simulink library "uavsimBlockset_Cularis"  (R2014b)
settings: Solver=ode45  StartTime=0.0  StopTime=10.0  RelTol=1e-3
undefined symbols (not defined in the file): aircraftmask_originNED_ECEF_rrm, aircraftmask_p0_NED_m, aircraftmask_phithetapsi0, aircraftmask_pqr0, aircraftmask_uvw0, fflib_degdegm2rrm, flat2lla, uavsim
libraries: uavsimBlockset_ServoHS55 x4, simulink_extras x1, uavsimBlockset_Cularis_Aerandpropulsion x1, uavsimblockset_SixDOFKinematics x1
settings Model: Creator=mstolle  LastModifiedBy=j.bolting

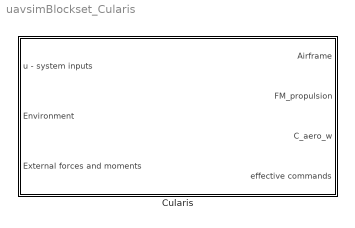
== system uavsimBlockset_Cularis ==
  Cularis : Subsystem  mask{mask_zagi_phithetapsi0=aircraftmask_phithetapsi0, mask_zagi_p0_ECEF_lla=fflib_degdegm2rrm(flat2lla(aircraftmask_p0_NED_m, rad2deg(aircraftmask_originNED_ECEF_rrm(1:2)), 0, aircraftmask_originNED_ECEF_rrm(3))), mask_zagi_originNED_ECEF_rrm=aircraftmask_originNED_ECEF_rrm, mask_zagi_pqr0=aircraftmask_pqr0, mask_zagi_uvw0=aircraftmask_uvw0, uavsim=uavsim}
      mask prompts: mask_zagi_phithetapsi0 "Initial euler angles [rad]"; mask_zagi_p0_ECEF_lla "Initial position ECEF [rad rad m]"; mask_zagi_originNED_ECEF_rrm "Origin NED frame, ECEF-WGS84, [rad rad m]"; mask_zagi_pqr0 "Initial body rotation rates [rad/s]"; mask_zagi_uvw0 "Initial velocity body frame [m/s]"; uavsim "Parameter set"
      mask Display: image(imread('images/cularis.png'),[.3, .3, .4, .4])

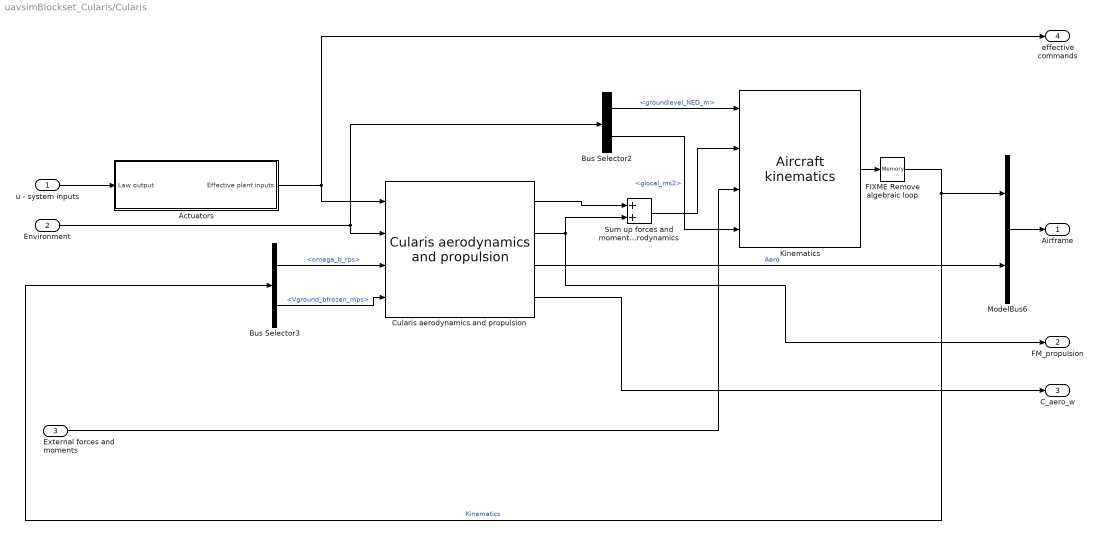
== system uavsimBlockset_Cularis/Cularis ==
  u - system inputs : Inport  OutDataTypeStr=Bus: CMD
  Environment : Inport  Port=2  OutDataTypeStr=Bus: Environment
  External forces and moments : Inport  Port=3
  Actuators : Subsystem  TreatAsAtomicUnit=on
  Bus Selector2 : BusSelector  OutputSignals=groundlevel_NED_m,glocal_ms2
  Bus Selector3 : BusSelector  OutputSignals=RotationalVelocity.omega_b_rps,Velocity.Vground_bfrozen_mps
  Cularis aerodynamics and propulsion : uavsimBlockset_Cularis_Aerandpropulsion/Cularis aerodynamics and propulsion  SystemSampleTime=-1
  FIXME Remove algebraic loop : Memory  X0=1e-6
  Kinematics : uavsimblockset_SixDOFKinematics/Aircraft kinematics  mask_inertia=uavsim.zagi.inertiaTensor  mask_mass=uavsim.zagi.mass  mask_P0_ECEF_rrm=mask_zagi_p0_ECEF_lla  mask_originNED_ECEF_rrm=mask_zagi_originNED_ECEF_rrm  mask_uvw0=mask_zagi_uvw0  mask_phithetapsi0=mask_zagi_phithetapsi0  mask_omega0=mask_zagi_pqr0
  ModelBus6 : BusCreator  Inputs=2  OutDataTypeStr=Bus: Airframe  NonVirtualBus=on
  Sum up forces and moments of engine and aircraft aerodynamics : Sum
  Airframe : Outport  OutDataTypeStr=Bus: Airframe
  FM_propulsion : Outport  Port=2
  C_aero_w : Outport  Port=3
  effective commands : Outport  Port=4  OutDataTypeStr=Bus: CMD
  wires:
  FIXME Remove algebraic loop/1 -> ModelBus6/1, Bus Selector3/1  "Kinematics"
  Actuators/1(Effective plant inputs) -> Cularis aerodynamics and propulsion/1, effective commands/1
  u - system inputs/1 -> Actuators/1(Law output)
  Bus Selector2/1 -> Kinematics/1  "<groundlevel_NED_m>"
  Bus Selector2/2 -> Kinematics/4  "<glocal_ms2>"
  Bus Selector3/1 -> Cularis aerodynamics and propulsion/3  "<omega_b_rps>"
  Bus Selector3/2 -> Cularis aerodynamics and propulsion/4  "<Vground_bfrozen_mps>"
  ModelBus6/1 -> Airframe/1
  Cularis aerodynamics and propulsion/3 -> ModelBus6/2  "Aero"
  Environment/1 -> Cularis aerodynamics and propulsion/2, Bus Selector2/1
  External forces and moments/1 -> Kinematics/3
  Cularis aerodynamics and propulsion/4 -> C_aero_w/1
  Cularis aerodynamics and propulsion/1 -> Sum up forces and moments of engine and aircraft aerodynamics/1
  Cularis aerodynamics and propulsion/2 -> FM_propulsion/1, Sum up forces and moments of engine and aircraft aerodynamics/2
  Sum up forces and moments of engine and aircraft aerodynamics/1 -> Kinematics/2
  Kinematics/1 -> FIXME Remove algebraic loop/1

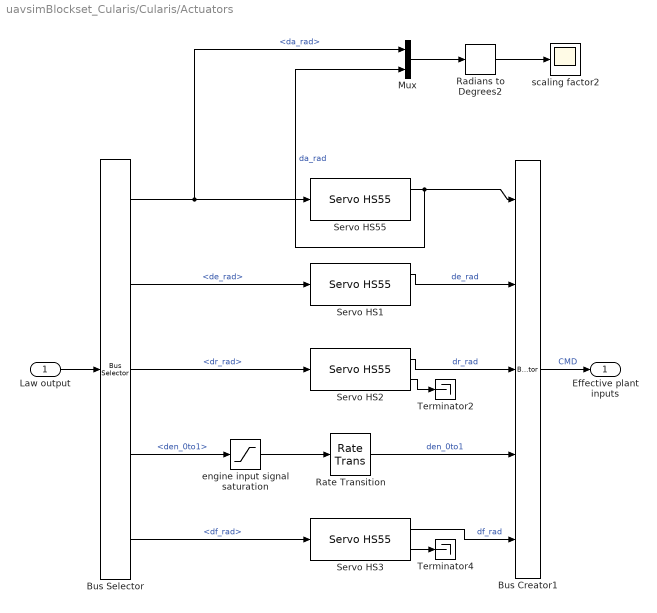
== system uavsimBlockset_Cularis/Cularis/Actuators ==
  Law output : Inport  OutDataTypeStr=Bus: CMD
  Bus Creator1 : BusCreator  Inputs=5  OutDataTypeStr=Bus: CMD  NonVirtualBus=on
  Bus Selector : BusSelector  OutputSignals=da_rad,de_rad,dr_rad,den_0to1,df_rad
  Mux : Mux  Inputs=2
  Radians to Degrees2 : simulink_extras/Transformations/Radians to Degrees
  Rate Transition : RateTransition  Integrity=off
  Servo HS1 : uavsimBlockset_ServoHS55/Servo HS55  deflectionLimits_rad=[deg2rad(-45) deg2rad(45)]  rateLimit_enabled=on  outputLimit_enabled=on  mask_initialPosition=uavsim.aircraftLibraryData.zagi.u0.de
  Servo HS2 : uavsimBlockset_ServoHS55/Servo HS55  deflectionLimits_rad=[deg2rad(-45) deg2rad(45)]  rateLimit_enabled=on  outputLimit_enabled=on  mask_initialPosition=uavsim.aircraftLibraryData.zagi.u0.dr
  Servo HS3 : uavsimBlockset_ServoHS55/Servo HS55  deflectionLimits_rad=[deg2rad(-10) deg2rad(90)]  rateLimit_enabled=on  outputLimit_enabled=on  mask_initialPosition=uavsim.aircraftLibraryData.zagi.u0.df
  Servo HS55 : uavsimBlockset_ServoHS55/Servo HS55  deflectionLimits_rad=[deg2rad(-45) deg2rad(45)]  rateLimit_enabled=on  outputLimit_enabled=on  mask_initialPosition=uavsim.aircraftLibraryData.zagi.u0.da
  Terminator2 : Terminator
  Terminator4 : Terminator
  engine input signal saturation : Saturate  UpperLimit=1  LowerLimit=0
  scaling factor2 : Scope
      settings: TimeRange=14  YMin=-30  YMax=60  SaveName=ScopeData40  MaxDataPoints=500000
  Effective plant inputs : Outport  OutDataTypeStr=Bus: CMD
  wires:
  Radians to Degrees2/1 -> scaling factor2/1
  Mux/1 -> Radians to Degrees2/1
  Servo HS3/2 -> Terminator4/1
  Servo HS2/2 -> Terminator2/1
  engine input signal saturation/1 -> Rate Transition/1
  Rate Transition/1 -> Bus Creator1/4  "den_0to1"
  Bus Selector/1 -> Servo HS55/1, Mux/1  "<da_rad>"
  Servo HS55/1 -> Bus Creator1/1, Mux/2  "da_rad"
  Servo HS1/1 -> Bus Creator1/2  "de_rad"
  Servo HS2/1 -> Bus Creator1/3  "dr_rad"
  Bus Selector/2 -> Servo HS1/1  "<de_rad>"
  Bus Selector/3 -> Servo HS2/1  "<dr_rad>"
  Bus Selector/4 -> engine input signal saturation/1  "<den_0to1>"
  Law output/1 -> Bus Selector/1
  Bus Creator1/1 -> Effective plant inputs/1  "CMD"
  Bus Selector/5 -> Servo HS3/1  "<df_rad>"
  Servo HS3/1 -> Bus Creator1/5  "df_rad"
